simulink model "PenduloInvertido"  (R2018a)
settings: Solver=ode4  StartTime=0.0  StopTime=150.0  FixedStep=0.1  RelTol=1e-3
values from neighbouring files (symbols this model uses):
  b = 0.05    [ParametrosPenduloInvertido.m]
  g = 9.81    [ParametrosPenduloInvertido.m]
  l = 0.45    [ParametrosPenduloInvertido.m]
  m = 0.5    [ParametrosPenduloInvertido.m]
  M = 2    [ParametrosPenduloInvertido.m]
libraries: vrlib x1
settings Model: Creator=Benjamin Nicolas  LastModifiedBy=Benjamin Nicolas

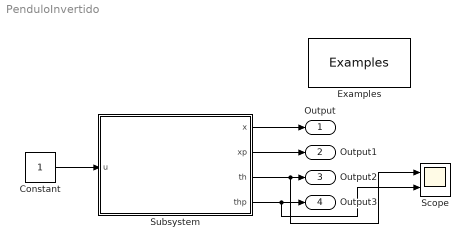
== system PenduloInvertido ==
  Constant : Constant
  Examples : vrlib/Examples
      settings: SourceProductName=Simulink 3D Animation  SourceProductBaseCode=VR
  Scope : Scope  NumInputPorts=2
  Subsystem : Subsystem
  Output : Outport
  Output1 : Outport  Port=2
  Output2 : Outport  Port=3
  Output3 : Outport  Port=4
  wires:
  Constant/1 -> Subsystem/1(u)
  Subsystem/1(x) -> Output/1
  Subsystem/2(xp) -> Output1/1
  Subsystem/3(th) -> Scope/1, Output2/1
  Subsystem/4(thp) -> Scope/2, Output3/1

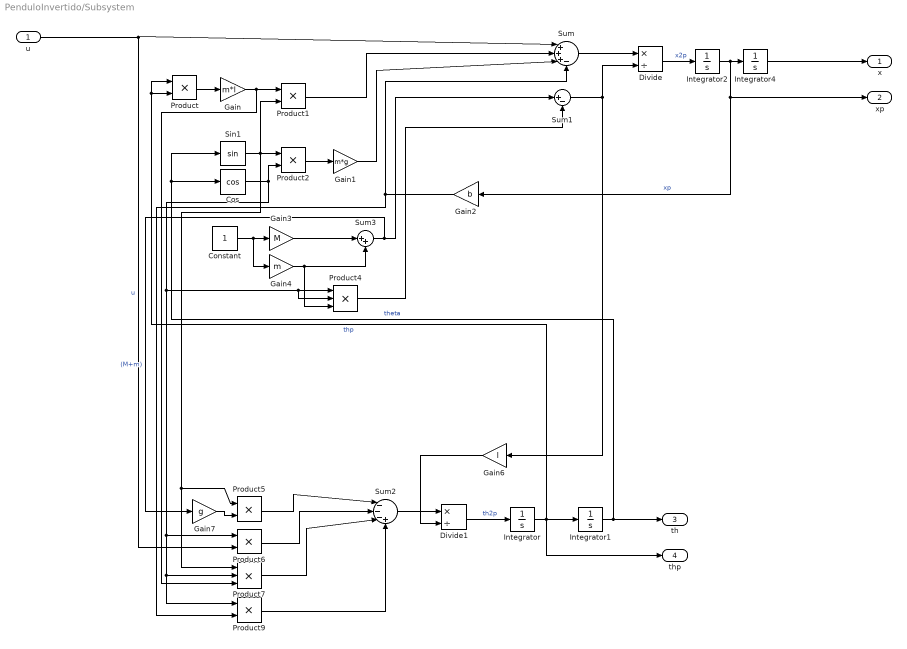
== system PenduloInvertido/Subsystem ==
  u : Inport
  Constant : Constant
  Cos : Trigonometry  Operator=cos
  Divide : Product  Inputs=*/
  Divide1 : Product  Inputs=*/
  Gain : Gain  Gain=m*l
  Gain1 : Gain  Gain=m*g
  Gain2 : Gain  Gain=b
  Gain3 : Gain  Gain=M
  Gain4 : Gain  Gain=m
  Gain6 : Gain  Gain=l
  Gain7 : Gain  Gain=g
  Integrator{,1..2,4} (4 alike) : Integrator  InitialCondition=pi/4
  Product{,1..2,5..6,9} (6 alike) : Product
  Product4 : Product  Inputs=3
  Product7 : Product  Inputs=3
  Sin1 : Trigonometry
  Sum : Sum  Inputs=|+++-
  Sum1 : Sum  Inputs=|+-
  Sum2 : Sum  Inputs=|---+
  Sum3 : Sum  Inputs=|++
  x : Outport
  xp : Outport  Port=2
  th : Outport  Port=3
  thp : Outport  Port=4
  wires:
  u/1 -> Sum/1, Product6/2  "u"
  Product2/1 -> Gain1/1
  Gain1/1 -> Sum/3
  Constant/1 -> Gain4/1, Gain3/1
  Sin1/1 -> Product1/2, Product7/1, Product5/1, Product2/1
  Integrator1/1 -> Sin1/1, Cos/1, th/1  "theta"
  Integrator2/1 -> Gain2/1, xp/1, Integrator4/1  "xp"
  Divide1/1 -> Integrator/1  "th2p"
  Integrator/1 -> Product/2, Product/1, thp/1, Integrator1/1  "thp"
  Product1/1 -> Sum/2
  Gain7/1 -> Product5/2
  Cos/1 -> Product9/1, Product7/2, Product6/1, Product4/2, Product4/1, Product2/2
  Sum1/1 -> Gain6/1, Divide/2
  Gain3/1 -> Sum3/1
  Divide/1 -> Integrator2/1  "x2p"
  Sum3/1 -> Gain7/1, Sum1/1  "(M+m)"
  Gain6/1 -> Divide1/2
  Product9/1 -> Sum2/4
  Gain2/1 -> Product9/2, Sum/4
  Product5/1 -> Sum2/1
  Sum2/1 -> Divide1/1
  Gain4/1 -> Product4/3, Sum3/2
  Product6/1 -> Sum2/2
  Integrator4/1 -> x/1
  Product4/1 -> Sum1/2
  Sum/1 -> Divide/1
  Product7/1 -> Sum2/3
  Gain/1 -> Product7/3, Product1/1
  Product/1 -> Gain/1
